simulink model "FCU_heat_exchanger"  (R2017a)
settings: Solver=VariableStepAuto  StartTime=0.0  StopTime=50000  RelTol=1e-3
settings Model: Creator=info  LastModifiedBy=info

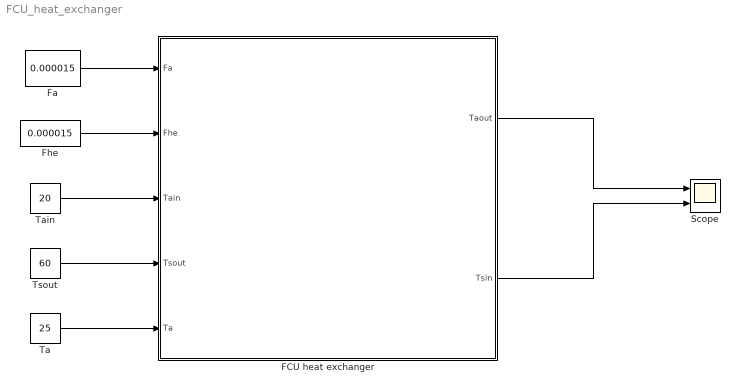
== system FCU_heat_exchanger ==
  FCU heat exchanger : Subsystem
      mask Display: image('heat_pump.PNG');
  Fa : Constant  Value=0.000015
  Fhe : Constant  Value=0.000015
  Scope : Scope  NumInputPorts=2
  Ta : Constant  Value=25
  Tain : Constant  Value=20
  Tsout : Constant  Value=60
  wires:
  Tsout/1 -> FCU heat exchanger/4("Tsout ")
  Tain/1 -> FCU heat exchanger/3("Tain ")
  Fhe/1 -> FCU heat exchanger/2(Fhe)
  Fa/1 -> FCU heat exchanger/1("Fa ")
  FCU heat exchanger/1("Taout ") -> Scope/1
  FCU heat exchanger/2("Tsin ") -> Scope/2
  Ta/1 -> FCU heat exchanger/5(Ta)

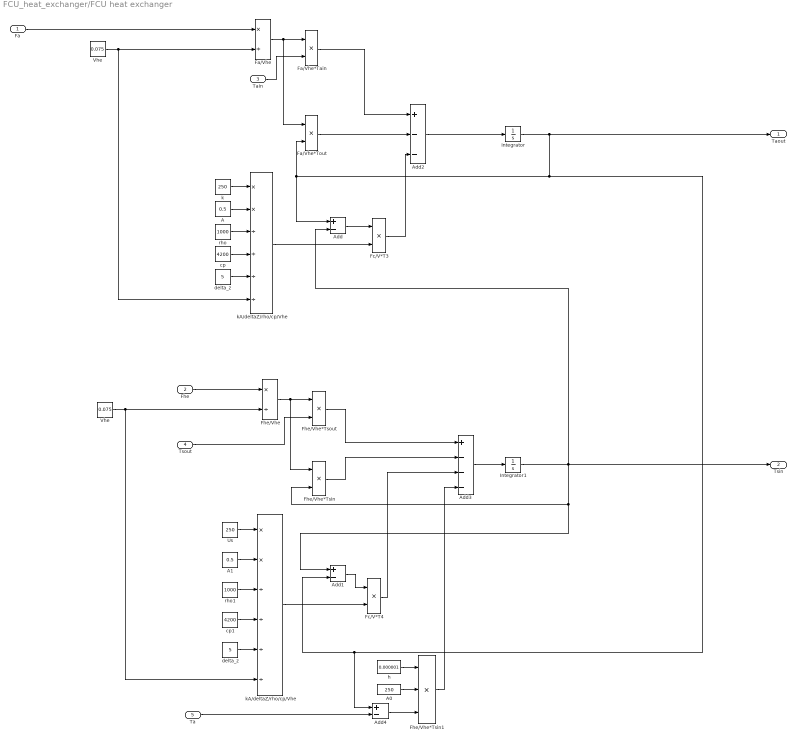
== system FCU_heat_exchanger/FCU heat exchanger ==
  "Fa " : Inport
  Fhe : Inport  Port=2
  "Tain " : Inport  Port=3
  "Tsout " : Inport  Port=4
  Ta : Inport  Port=5
  A : Constant  Value=0.5
  A0 : Constant  Value=250
  A1 : Constant  Value=0.5
  Add : Sum  Inputs=+-
  Add1 : Sum  Inputs=+-
  Add2 : Sum  Inputs=+--
  Add3 : Sum  Inputs=+---
  Add4 : Sum  Inputs=+-
  Fa/Vhe : Product  Inputs=*/
  Fa/Vhe*Tain : Product  Inputs=**
  Fa/Vhe*Tout : Product  Inputs=**
  Fc/V*T3 : Product  Inputs=**
  Fc/V*T4 : Product  Inputs=**
  Fhe/Vhe : Product  Inputs=*/
  Fhe/Vhe*Tsin : Product  Inputs=**
  Fhe/Vhe*Tsin1 : Product  Inputs=***
  Fhe/Vhe*Tsout : Product  Inputs=**
  Integrator : Integrator  InitialCondition=16.87
  Integrator1 : Integrator  InitialCondition=10
  "Us    " : Constant  Value=250
  Vhe : Constant  Value=0.075
  "Vhe " : Constant  Value=0.075
  cp : Constant  Value=4200
  cp1 : Constant  Value=4200
  delta_z : Constant  Value=5
  "delta_z " : Constant  Value=5
  h : Constant  Value=0.000001
  k : Constant  Value=250
  kA/deltaZ/rho/cp/Vhe : Product  Inputs=**////
  "kA/deltaZ/rho/cp/Vhe " : Product  Inputs=**////
  rho : Constant  Value=1000
  rho1 : Constant  Value=1000
  "Taout " : Outport
  "Tsin " : Outport  Port=2
  wires:
  Vhe/1 -> kA/deltaZ/rho/cp/Vhe/6, Fa/Vhe/2
  "Us    "/1 -> "kA/deltaZ/rho/cp/Vhe "/1
  Integrator1/1 -> Add1/1, Fhe/Vhe*Tsin/2, "Tsin "/1, Add/2
  "Tsout "/1 -> Fhe/Vhe*Tsout/2
  "Fa "/1 -> Fa/Vhe/1
  Fa/Vhe/1 -> Fa/Vhe*Tout/1, Fa/Vhe*Tain/1
  rho/1 -> kA/deltaZ/rho/cp/Vhe/3
  cp1/1 -> "kA/deltaZ/rho/cp/Vhe "/4
  A1/1 -> "kA/deltaZ/rho/cp/Vhe "/2
  Integrator/1 -> Add4/1, Add1/2, Fa/Vhe*Tout/2, Add/1, "Taout "/1
  k/1 -> kA/deltaZ/rho/cp/Vhe/1
  "Tain "/1 -> Fa/Vhe*Tain/2
  rho1/1 -> "kA/deltaZ/rho/cp/Vhe "/3
  Fhe/Vhe/1 -> Fhe/Vhe*Tsout/1, Fhe/Vhe*Tsin/1
  "Vhe "/1 -> "kA/deltaZ/rho/cp/Vhe "/6, Fhe/Vhe/2
  Fhe/1 -> Fhe/Vhe/1
  cp/1 -> kA/deltaZ/rho/cp/Vhe/4
  A/1 -> kA/deltaZ/rho/cp/Vhe/2
  Fa/Vhe*Tain/1 -> Add2/1
  Add2/1 -> Integrator/1
  kA/deltaZ/rho/cp/Vhe/1 -> Fc/V*T3/2
  Fc/V*T3/1 -> Add2/3
  Fhe/Vhe*Tsout/1 -> Add3/1
  Add3/1 -> Integrator1/1
  Add/1 -> Fc/V*T3/1
  Fa/Vhe*Tout/1 -> Add2/2
  Fhe/Vhe*Tsin/1 -> Add3/2
  Fc/V*T4/1 -> Add3/3
  "kA/deltaZ/rho/cp/Vhe "/1 -> Fc/V*T4/2
  Add1/1 -> Fc/V*T4/1
  delta_z/1 -> kA/deltaZ/rho/cp/Vhe/5
  "delta_z "/1 -> "kA/deltaZ/rho/cp/Vhe "/5
  Fhe/Vhe*Tsin1/1 -> Add3/4
  Ta/1 -> Add4/2
  Add4/1 -> Fhe/Vhe*Tsin1/3
  h/1 -> Fhe/Vhe*Tsin1/1
  A0/1 -> Fhe/Vhe*Tsin1/2
